simulink model "Demonstration2"  (R2025a)
settings: Solver=VariableStepAuto  StartTime=0.0  StopTime=3  MaxStep=0.001  RelTol=1e-3
InitFcn:
  | clear all;
  | 
  | % Bauteilgrößen
  | R = 1e3;
  | L = 10e-3;
  | C1 = 100e-9;
  | C2 = 1e-6;
  | 
  | % weitere physikalische Größen
  | k  = 1.380649e-23;
  | e  = 1.602176634e-19;
  | T_C = 25;
  | T_K = 273.15;
  | T = T_C + T_K;
  | UT = k*T/e;
  | IS = 10e-9;
  | 
  | % Reglermatrix für EAL von U1
  | G_U1 = [50 10];
  | 
  | % Reglermatrix für EAL von U2 und IL
  | G_U2 = 5;
  | G_IL = 5;
settings Model: Creator=richa  LastModifiedBy=richa

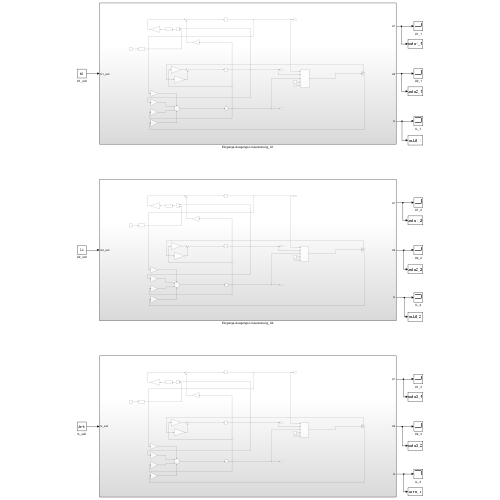
[thumbnail: Simulink's stored preview of the top-level diagram]
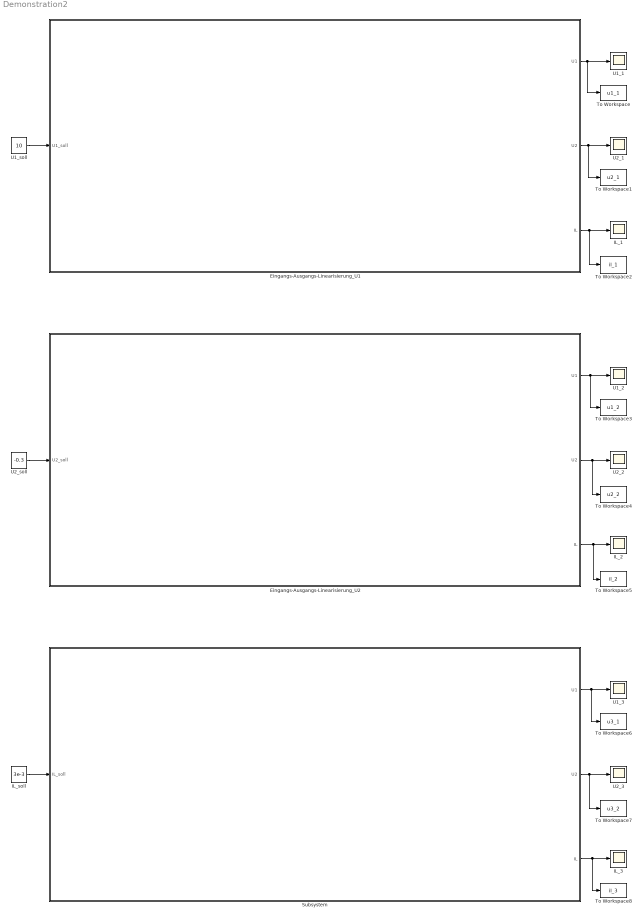
== system Demonstration2 ==
  Eingangs-Ausgangs-Linearisierung_U1 : Subsystem
  Eingangs-Ausgangs-Linearisierung_U2 : Subsystem
  IL_1 : Scope
      settings: ActiveDisplayYMinimum=-5.5973212986714648E-7  ActiveDisplayYMaximum=3.6443842769786703E-6  DataLoggingVariableName=ScopeData2
  IL_2 : Scope
      settings: ActiveDisplayYMinimum=-0.00012438633420110688  ActiveDisplayYMaximum=0.0013985306041250391  DataLoggingVariableName=ScopeData3
  IL_3 : Scope
      settings: ActiveDisplayYMinimum=-0.00037499988682156339  ActiveDisplayYMaximum=0.0033749989813940716  DataLoggingVariableName=ScopeData6
  IL_soll : Constant  Value=3e-3
  Subsystem : Subsystem
  To Workspace : ToWorkspace  VariableName=u1_1  SaveFormat=Structure With Time  SampleTime=-1
  To Workspace1 : ToWorkspace  VariableName=u2_1  SaveFormat=Structure With Time  SampleTime=-1
  To Workspace2 : ToWorkspace  VariableName=il_1  SaveFormat=Structure With Time  SampleTime=-1
  To Workspace3 : ToWorkspace  VariableName=u1_2  SaveFormat=Structure With Time  SampleTime=-1
  To Workspace4 : ToWorkspace  VariableName=u2_2  SaveFormat=Structure With Time  SampleTime=-1
  To Workspace5 : ToWorkspace  VariableName=il_2  SaveFormat=Structure With Time  SampleTime=-1
  To Workspace6 : ToWorkspace  VariableName=u3_1  SaveFormat=Structure With Time  SampleTime=-1
  To Workspace7 : ToWorkspace  VariableName=u3_2  SaveFormat=Structure With Time  SampleTime=-1
  To Workspace8 : ToWorkspace  VariableName=il_3  SaveFormat=Structure With Time  SampleTime=-1
  U1_1 : Scope
      settings: ActiveDisplayYMinimum=-1.3040286511284684  ActiveDisplayYMaximum=11.736158320813463
  U1_2 : Scope
      settings: ActiveDisplayYMinimum=-1.0096110625550929  ActiveDisplayYMaximum=0.30774593097452607  DataLoggingVariableName=ScopeData4
  U1_3 : Scope
      settings: ActiveDisplayYMinimum=-10500.000248326513  ActiveDisplayYMaximum=94500.002234938627  DataLoggingVariableName=ScopeData7
  U1_soll : Constant  Value=10
  U2_1 : Scope
      settings: ActiveDisplayYMinimum=-0.1534417280698547  ActiveDisplayYMaximum=1.3809723924981259
  U2_2 : Scope
      settings: ActiveDisplayYMinimum=-0.337499896757956  ActiveDisplayYMaximum=0.037499988528661772  DataLoggingVariableName=ScopeData5
  U2_3 : Scope
      settings: ActiveDisplayYMinimum=-1050.000026886564  ActiveDisplayYMaximum=9450.0002419790781  DataLoggingVariableName=ScopeData8
  U2_soll : Constant  Value=-0.3
  wires:
  Eingangs-Ausgangs-Linearisierung_U1/1(U1) -> U1_1/1, To Workspace/1
  Eingangs-Ausgangs-Linearisierung_U1/2(U2) -> To Workspace1/1, U2_1/1
  Eingangs-Ausgangs-Linearisierung_U1/3(IL) -> To Workspace2/1, IL_1/1
  U1_soll/1 -> Eingangs-Ausgangs-Linearisierung_U1/1(U1_soll)
  Eingangs-Ausgangs-Linearisierung_U2/1(U1) -> To Workspace3/1, U1_2/1
  Eingangs-Ausgangs-Linearisierung_U2/2(U2) -> To Workspace4/1, U2_2/1
  Eingangs-Ausgangs-Linearisierung_U2/3(IL) -> To Workspace5/1, IL_2/1
  U2_soll/1 -> Eingangs-Ausgangs-Linearisierung_U2/1(U2_soll)
  Subsystem/2(U2) -> To Workspace7/1, U2_3/1
  Subsystem/1(U1) -> To Workspace6/1, U1_3/1
  Subsystem/3(IL) -> To Workspace8/1, IL_3/1
  IL_soll/1 -> Subsystem/1(IL_soll)

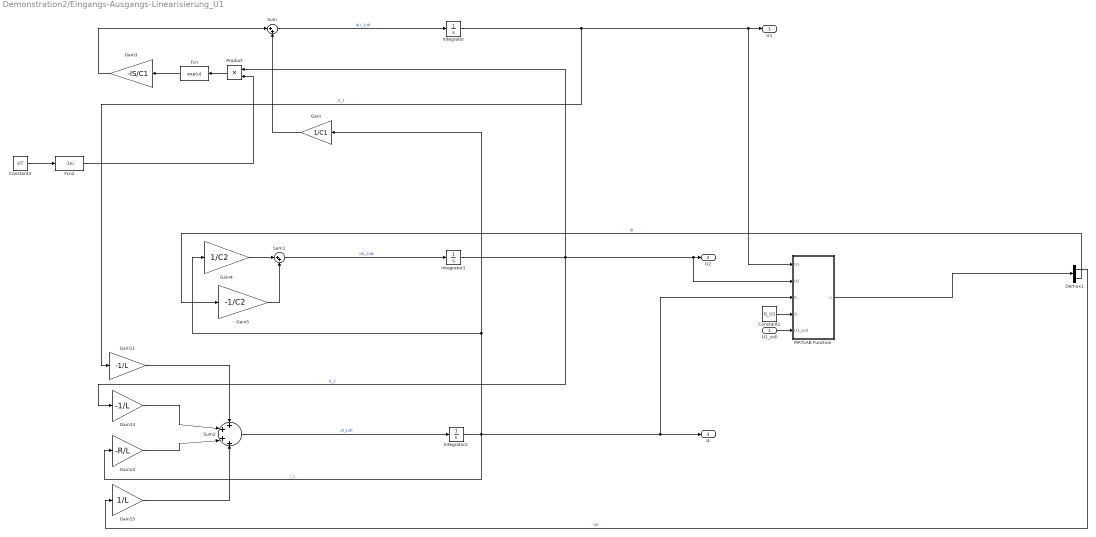
== system Demonstration2/Eingangs-Ausgangs-Linearisierung_U1 ==
  U1_soll : Inport
  Constant1 : Constant  Value=G_U1
  Constant3 : Constant  Value=UT
  Demux1 : Demux  Outputs=2
  Fcn : Fcn  Expr=exp(u)
  Fcn2 : Fcn  Expr=-1/u
  Gain : Gain  Gain=1/C1
  Gain11 : Gain  Gain=-1/L
  Gain13 : Gain  Gain=-1/L
  Gain14 : Gain  Gain=-R/L
  Gain15 : Gain  Gain=1/L
  Gain3 : Gain  Gain=-IS/C1
  Gain4 : Gain  Gain=1/C2
  Gain5 : Gain  Gain=-1/C2
  Integrator : Integrator
  Integrator1 : Integrator
  Integrator2 : Integrator
  MATLAB Function : MATLAB Function  TreatAsAtomicUnit=on
  Product : Product
  Sum : Sum  Inputs=|++
  Sum1 : Sum  Inputs=|++
  Sum2 : Sum  Inputs=++++
  U1 : Outport
  U2 : Outport  Port=2
  IL : Outport  Port=3
  wires:
  Gain4/1 -> Sum1/1
  Gain11/1 -> Sum2/1
  Fcn2/1 -> Product/2
  Gain/1 -> Sum/2
  Gain13/1 -> Sum2/2
  Gain5/1 -> Sum1/2
  Integrator1/1 -> MATLAB Function/2(U2), U2/1, Product/1, Gain13/1  "U_2"
  Gain3/1 -> Sum/1
  Sum1/1 -> Integrator1/1  "dU_2/dt"
  Integrator/1 -> MATLAB Function/1(U1), U1/1, Gain11/1  "U_1"
  Constant3/1 -> Fcn2/1
  Product/1 -> Fcn/1
  Gain14/1 -> Sum2/3
  Sum/1 -> Integrator/1  "dU_1/dt"
  Fcn/1 -> Gain3/1
  Gain15/1 -> Sum2/4
  Sum2/1 -> Integrator2/1  "dI_L/dt"
  Integrator2/1 -> MATLAB Function/3(IL), IL/1, Gain14/1, Gain/1, Gain4/1  "I_L"
  Demux1/1 -> Gain15/1  "U0"
  Demux1/2 -> Gain5/1  "I0"
  MATLAB Function/1(u) -> Demux1/1
  Constant1/1 -> MATLAB Function/4(G)
  U1_soll/1 -> MATLAB Function/5(U1_soll)

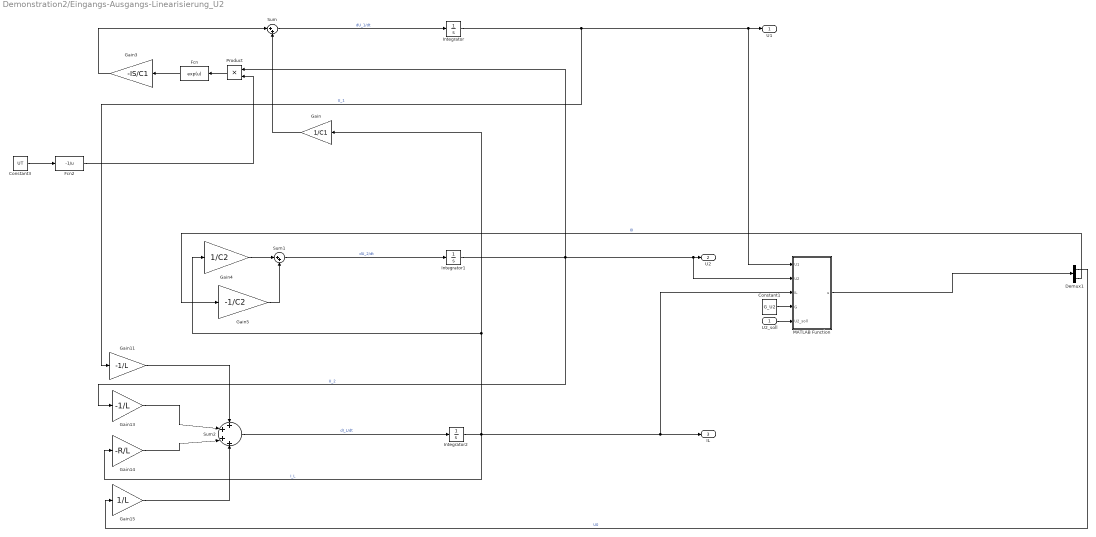
== system Demonstration2/Eingangs-Ausgangs-Linearisierung_U2 ==
  U2_soll : Inport
  Constant1 : Constant  Value=G_U2
  Constant3 : Constant  Value=UT
  Demux1 : Demux  Outputs=2
  Fcn : Fcn  Expr=exp(u)
  Fcn2 : Fcn  Expr=-1/u
  Gain : Gain  Gain=1/C1
  Gain11 : Gain  Gain=-1/L
  Gain13 : Gain  Gain=-1/L
  Gain14 : Gain  Gain=-R/L
  Gain15 : Gain  Gain=1/L
  Gain3 : Gain  Gain=-IS/C1
  Gain4 : Gain  Gain=1/C2
  Gain5 : Gain  Gain=-1/C2
  Integrator : Integrator
  Integrator1 : Integrator
  Integrator2 : Integrator
  MATLAB Function : MATLAB Function  TreatAsAtomicUnit=on
  Product : Product
  Sum : Sum  Inputs=|++
  Sum1 : Sum  Inputs=|++
  Sum2 : Sum  Inputs=++++
  U1 : Outport
  U2 : Outport  Port=2
  IL : Outport  Port=3
  wires:
  Gain4/1 -> Sum1/1
  Gain11/1 -> Sum2/1
  Fcn2/1 -> Product/2
  Gain/1 -> Sum/2
  Gain13/1 -> Sum2/2
  Gain5/1 -> Sum1/2
  Integrator1/1 -> MATLAB Function/2(U2), U2/1, Product/1, Gain13/1  "U_2"
  Gain3/1 -> Sum/1
  Sum1/1 -> Integrator1/1  "dU_2/dt"
  Integrator/1 -> MATLAB Function/1(U1), U1/1, Gain11/1  "U_1"
  Constant3/1 -> Fcn2/1
  Product/1 -> Fcn/1
  Gain14/1 -> Sum2/3
  Sum/1 -> Integrator/1  "dU_1/dt"
  Fcn/1 -> Gain3/1
  Gain15/1 -> Sum2/4
  Sum2/1 -> Integrator2/1  "dI_L/dt"
  Integrator2/1 -> MATLAB Function/3(IL), IL/1, Gain14/1, Gain/1, Gain4/1  "I_L"
  Demux1/1 -> Gain15/1  "U0"
  Demux1/2 -> Gain5/1  "I0"
  MATLAB Function/1(u) -> Demux1/1
  Constant1/1 -> MATLAB Function/4(G)
  U2_soll/1 -> MATLAB Function/5(U2_soll)

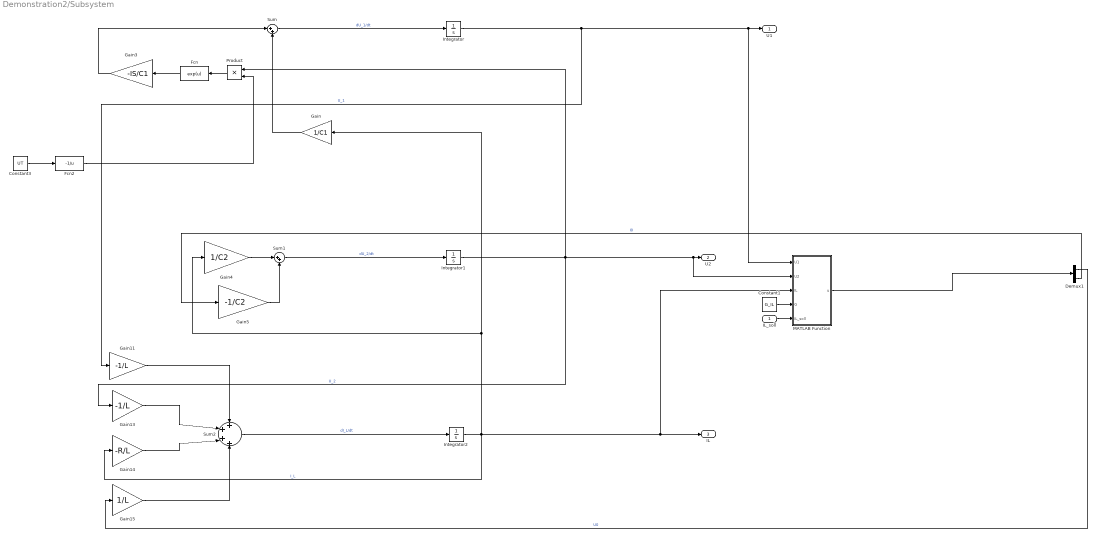
== system Demonstration2/Subsystem ==
  IL_soll : Inport
  Constant1 : Constant  Value=G_IL
  Constant3 : Constant  Value=UT
  Demux1 : Demux  Outputs=2
  Fcn : Fcn  Expr=exp(u)
  Fcn2 : Fcn  Expr=-1/u
  Gain : Gain  Gain=1/C1
  Gain11 : Gain  Gain=-1/L
  Gain13 : Gain  Gain=-1/L
  Gain14 : Gain  Gain=-R/L
  Gain15 : Gain  Gain=1/L
  Gain3 : Gain  Gain=-IS/C1
  Gain4 : Gain  Gain=1/C2
  Gain5 : Gain  Gain=-1/C2
  Integrator : Integrator
  Integrator1 : Integrator
  Integrator2 : Integrator
  MATLAB Function : MATLAB Function  TreatAsAtomicUnit=on
  Product : Product
  Sum : Sum  Inputs=|++
  Sum1 : Sum  Inputs=|++
  Sum2 : Sum  Inputs=++++
  U1 : Outport
  U2 : Outport  Port=2
  IL : Outport  Port=3
  wires:
  Gain4/1 -> Sum1/1
  Gain11/1 -> Sum2/1
  Fcn2/1 -> Product/2
  Gain/1 -> Sum/2
  Gain13/1 -> Sum2/2
  Gain5/1 -> Sum1/2
  Integrator1/1 -> MATLAB Function/2(U2), U2/1, Product/1, Gain13/1  "U_2"
  Gain3/1 -> Sum/1
  Sum1/1 -> Integrator1/1  "dU_2/dt"
  Integrator/1 -> MATLAB Function/1(U1), U1/1, Gain11/1  "U_1"
  Constant3/1 -> Fcn2/1
  Product/1 -> Fcn/1
  Gain14/1 -> Sum2/3
  Sum/1 -> Integrator/1  "dU_1/dt"
  Fcn/1 -> Gain3/1
  Gain15/1 -> Sum2/4
  Sum2/1 -> Integrator2/1  "dI_L/dt"
  Integrator2/1 -> MATLAB Function/3(IL), IL/1, Gain14/1, Gain/1, Gain4/1  "I_L"
  Demux1/1 -> Gain15/1  "U0"
  Demux1/2 -> Gain5/1  "I0"
  MATLAB Function/1(u) -> Demux1/1
  Constant1/1 -> MATLAB Function/4(G)
  IL_soll/1 -> MATLAB Function/5(IL_soll)

== matlab function Demonstration2/Eingangs-Ausgangs-Linearisierung_U2/MATLAB Function ==
  data: U1 input; u output; U2 input; IL input; G input; U2_soll input
function u = fcn(U1, U2, IL, G, U2_soll)
    
    % z = phi(x) = phi(U1, U2, IL)
    z = U2;
    
    % v = - G * (z - z_ref)
    v = -G * (z - U2_soll);
    
    % u = alpha^-1 * (v - beta)
    u =  [0; -1/1000000] * (v - 1000000*IL);

end

== matlab function Demonstration2/Eingangs-Ausgangs-Linearisierung_U1/MATLAB Function ==
  data: U1 input; u output; U2 input; IL input; G input; U1_soll input
function u = fcn(U1, U2, IL, G, U1_soll)
    
    % z = phi(x) = phi(U1, U2, IL)
    z = [U1; 10000000*IL - exp(-(144115188075855872*U2)/3702690872189095)/10];
    
    % v = - G * (z - z_ref)
    v = - G(1)*(z(1) - U1_soll) - G(2)*z(2);
    
    % u = alpha^-1 * (v - beta)
    u = [1000000000/((8307674973655724205648794126752153600000000*exp(-(144115188075855872*U2)/3702690872189095)*exp(-(144115188075855872*conj(U2))/3702690872189095))/548396787799697641796697476761 + 1000000000000000000); -(2882303761517117440000*exp(-(144115188075855872*conj(U2))/3702690872189095))/(740538174437819*((8307674973655724205648794126752153600000000*exp(-(144115188075855872*U2)/3702690872189095)*exp(-(144115188075855872*conj(U2))/3702690872189095))/548396787799697641796697476761 + 1000000000000000000))] * (v - ((2882303761517117440000*IL*exp(-(144115188075855872*U2)/3702690872189095))/740538174437819 - 1000000000*U1 - 1000000000*U2 - 1000000000000*IL));

end

== matlab function Demonstration2/Subsystem/MATLAB Function ==
  data: U1 input; u output; U2 input; IL input; G input; IL_soll input
function u = fcn(U1, U2, IL, G, IL_soll)
    
    % z = phi(x) = phi(U1, U2, IL)
    z = IL;
    
    % v = - G * (z - z_ref)
    v = -G * (z - IL_soll);
    
    % u = alpha^-1 * (v - beta)
    u =  [0.01; 0] * (v - (- 100000*IL - 100*U1 - 100*U2));

end
